simulink model "fw_att_control"  (R2024b)
settings: Solver=FixedStepAuto  StartTime=0.0  StopTime=10.0  FixedStep=0.005  RelTol=1e-3
undefined symbols (not defined in the file): DiscIntNeverNeededParam, FW_ACRO_X_MAX, FW_ACRO_Y_MAX, FW_ACRO_Z_MAX, FW_AIRSPD_MAX, FW_AIRSPD_STALL, FW_AIRSPD_TRIM, FW_ARSP_MODE, FW_ARSP_SCALE_EN, FW_BAT_SCALE_EN, FW_DTRIM_P_VMAX, FW_DTRIM_P_VMIN, FW_DTRIM_R_VMAX, FW_DTRIM_R_VMIN, FW_DTRIM_Y_VMAX, FW_DTRIM_Y_VMIN, FW_FLAPERON_SCL, FW_FLAPS_LND_SCL, FW_FLAPS_SCL, FW_FLAPS_TO_SCL, FW_MAN_P_MAX, FW_MAN_P_SC, FW_MAN_R_MAX, FW_MAN_R_SC, FW_MAN_Y_SC, FW_P_RMAX_NEG, FW_P_RMAX_POS, FW_P_TC, FW_PR_FF, FW_PR_IMAX, FW_PR_P, FW_PSP_OFF, FW_R_RMAX, FW_R_TC, FW_RLL_TO_YAW_FF, FW_RR_FF, FW_RR_IMAX, FW_RR_P, FW_W_RMAX, FW_WR_FF, FW_WR_IMAX, FW_WR_P, FW_Y_RMAX, FW_YR_FF, FW_YR_IMAX, FW_YR_P, TRIM_PITCH, TRIM_ROLL, TRIM_YAW
libraries: aerolibconvert2 x5, sharedtransform x2
settings Model: DataDictionary=nextpilot_datadict.sldd  Creator=CETCA  LastModifiedBy=CETCA
settings OptimizationCC: DefaultUnderspecifiedDataType=single
settings DebuggingCC: ParamPrecisionLossAbsoluteDiffThreshold=eps

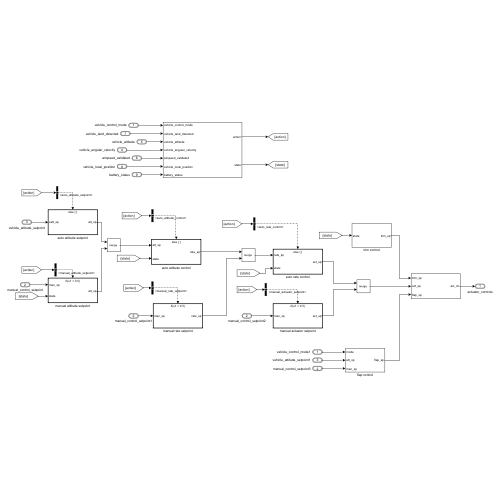
[thumbnail: Simulink's stored preview of the top-level diagram]
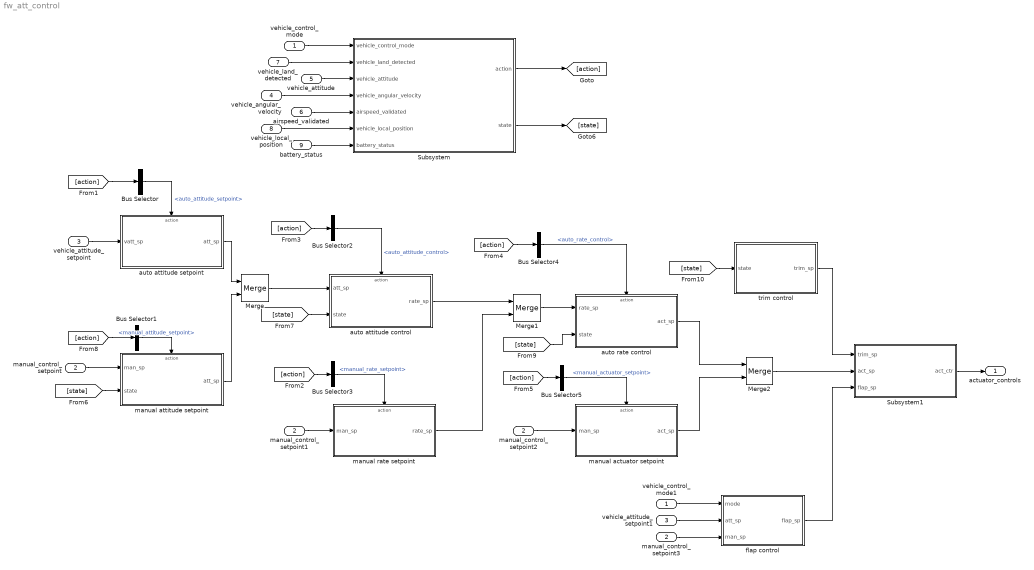
== system fw_att_control ==
  vehicle_control_mode : Inport  OutDataTypeStr=Bus: vehicle_control_mode_s
  manual_control_setpoint : Inport  Port=2  OutDataTypeStr=Bus: manual_control_setpoint_s
  vehicle_attitude_setpoint : Inport  Port=3  OutDataTypeStr=Bus:vehicle_attitude_setpoint_s
  vehicle_angular_velocity : Inport  Port=4  OutDataTypeStr=Bus: vehicle_angular_velocity_s
  vehicle_attitude : Inport  Port=5  OutDataTypeStr=Bus: vehicle_attitude_s
  airspeed_validated : Inport  Port=6  OutDataTypeStr=Bus: airspeed_validated_s
  vehicle_land_detected : Inport  Port=7  OutDataTypeStr=Bus: vehicle_land_detected_s
  vehicle_local_position : Inport  Port=8  OutDataTypeStr=Bus: vehicle_local_position_s
  battery_status : Inport  Port=9  OutDataTypeStr=Bus: battery_status_s
  Bus Selector : BusSelector  OutputSignals=auto_attitude_setpoint
  Bus Selector1 : BusSelector  OutputSignals=manual_attitude_setpoint
  Bus Selector2 : BusSelector  OutputSignals=auto_attitude_control
  Bus Selector3 : BusSelector  OutputSignals=manual_rate_setpoint
  Bus Selector4 : BusSelector  OutputSignals=auto_rate_control
  Bus Selector5 : BusSelector  OutputSignals=manual_actuator_setpoint
  Merge : Merge
  Merge1 : Merge
  Merge2 : Merge
  Subsystem : Subsystem
  Subsystem1 : Subsystem
  auto attitude control : Subsystem
  auto attitude setpoint : Subsystem
  auto rate control : Subsystem
  flap control : Subsystem
  manual actuator setpoint : Subsystem
  manual attitude setpoint : Subsystem
  manual rate setpoint : Subsystem
  manual_control_setpoint1 : InportShadow  Port=2  OutDataTypeStr=Bus: manual_control_setpoint_s
  manual_control_setpoint2 : InportShadow  Port=2  OutDataTypeStr=Bus: manual_control_setpoint_s
  manual_control_setpoint3 : InportShadow  Port=2  OutDataTypeStr=Bus: manual_control_setpoint_s
  trim control : Subsystem
  vehicle_attitude_setpoint1 : InportShadow  Port=3  OutDataTypeStr=Bus:vehicle_attitude_setpoint_s
  vehicle_control_mode1 : InportShadow  OutDataTypeStr=Bus: vehicle_control_mode_s
  actuator_controls : Outport  OutDataTypeStr=Bus: actuator_controls_s
  wires:
  manual_control_setpoint/1 -> manual attitude setpoint/1(man_sp)
  vehicle_attitude_setpoint/1 -> auto attitude setpoint/1(vatt_sp)
  Merge/1 -> auto attitude control/1(att_sp)
  auto attitude control/1(rate_sp) -> Merge1/1
  manual rate setpoint/1(rate_sp) -> Merge1/2
  Merge1/1 -> auto rate control/1(rate_sp)
  auto rate control/1(act_sp) -> Merge2/1
  manual actuator setpoint/1(act_sp) -> Merge2/2
  Bus Selector1/1 -> manual attitude setpoint/Action  "<manual_attitude_setpoint>"
  [action] -> Bus Selector/1
  Bus Selector3/1 -> manual rate setpoint/Action  "<manual_rate_setpoint>"
  Bus Selector2/1 -> auto attitude control/Action  "<auto_attitude_control>"
  Bus Selector5/1 -> manual actuator setpoint/Action  "<manual_actuator_setpoint>"
  Bus Selector4/1 -> auto rate control/Action  "<auto_rate_control>"
  vehicle_control_mode/1 -> Subsystem/1(vehicle_control_mode)
  manual_control_setpoint1/1 -> manual rate setpoint/1(man_sp)
  manual_control_setpoint2/1 -> manual actuator setpoint/1(man_sp)
  Subsystem/1(action) -> [action]
  vehicle_land_detected/1 -> Subsystem/2(vehicle_land_detected)
  airspeed_validated/1 -> Subsystem/5(airspeed_validated)
  vehicle_angular_velocity/1 -> Subsystem/4(vehicle_angular_velocity)
  vehicle_attitude/1 -> Subsystem/3(vehicle_attitude)
  Subsystem/2(state) -> [state]
  [state] -> manual attitude setpoint/2(state)
  vehicle_local_position/1 -> Subsystem/6(vehicle_local_position)
  [state] -> auto attitude control/2(state)
  manual attitude setpoint/1(att_sp) -> Merge/2
  auto attitude setpoint/1(att_sp) -> Merge/1
  Bus Selector/1 -> auto attitude setpoint/Action  "<auto_attitude_setpoint>"
  [action] -> Bus Selector1/1
  [action] -> Bus Selector2/1
  [action] -> Bus Selector3/1
  [action] -> Bus Selector4/1
  [action] -> Bus Selector5/1
  [state] -> auto rate control/2(state)
  battery_status/1 -> Subsystem/7(battery_status)
  Merge2/1 -> Subsystem1/2(act_sp)
  vehicle_attitude_setpoint1/1 -> flap control/2(att_sp)
  manual_control_setpoint3/1 -> flap control/3(man_sp)
  vehicle_control_mode1/1 -> flap control/1(mode)
  flap control/1(flap_sp) -> Subsystem1/3(flap_sp)
  Subsystem1/1(act_ctr) -> actuator_controls/1
  [state] -> trim control/1(state)
  trim control/1(trim_sp) -> Subsystem1/1(trim_sp)

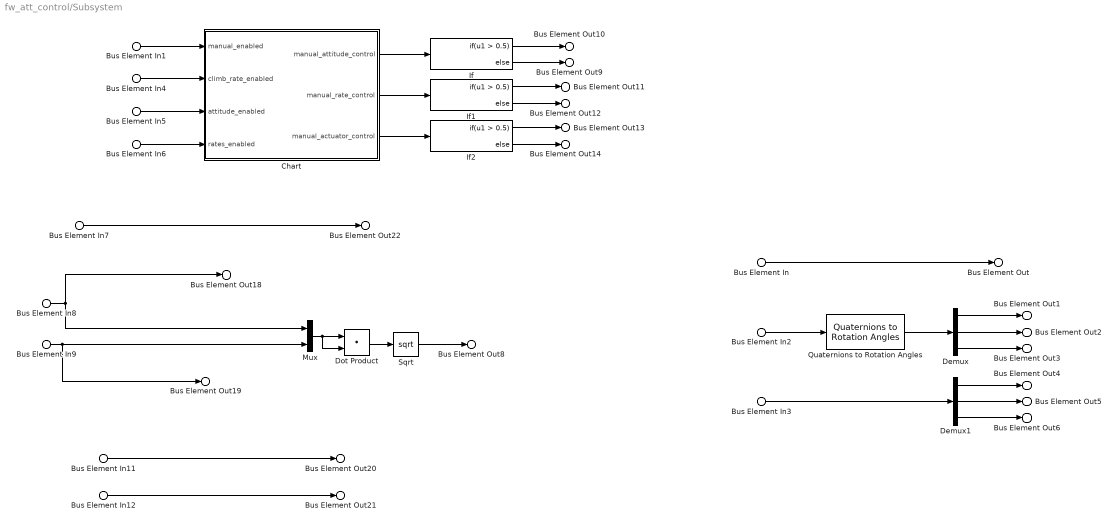
== system fw_att_control/Subsystem ==
  Bus Element In1 : Inport  PortName=vehicle_control_mode  Element=flag_control_manual_enabled
  Bus Element In4 : Inport  PortName=vehicle_control_mode  Element=flag_control_climb_rate_enabled
  Bus Element In5 : Inport  PortName=vehicle_control_mode  Element=flag_control_attitude_enabled
  Bus Element In6 : Inport  PortName=vehicle_control_mode  Element=flag_control_rates_enabled
  Bus Element In : Inport  Port=2  PortName=vehicle_land_detected  Element=landed
  Bus Element In2 : Inport  Port=3  PortName=vehicle_attitude  Element=q
  Bus Element In3 : Inport  Port=4  PortName=vehicle_angular_velocity  Element=xyz
  Bus Element In7 : Inport  Port=5  PortName=airspeed_validated  Element=calibrated_airspeed_m_s
  Bus Element In8 : Inport  Port=6  PortName=vehicle_local_position  Element=vx
  Bus Element In9 : Inport  Port=6  PortName=vehicle_local_position  Element=vy
  Bus Element In11 : Inport  Port=7  PortName=battery_status  Element=connected
  Bus Element In12 : Inport  Port=7  PortName=battery_status  Element=scale
  Chart : Stateflow chart  TreatAsAtomicUnit=on
  Demux : Demux  Outputs=3
  Demux1 : Demux  Outputs=3
  Dot Product : DotProduct  OutDataTypeStr=Inherit: Inherit via internal rule
  If : If  IfExpression=u1 > 0.5
  If1 : If  IfExpression=u1 > 0.5
  If2 : If  IfExpression=u1 > 0.5
  Mux : Mux  Inputs=2
  Quaternions to Rotation Angles : sharedtransform/Quaternions to Rotation Angles  rotationOrder=ZYX  aMode=aMode
  Sqrt : Sqrt
  Bus Element Out10 : Outport  PortName=action  Element=manual_attitude_setpoint
  Bus Element Out9 : Outport  PortName=action  Element=auto_attitude_setpoint
  Bus Element Out11 : Outport  PortName=action  Element=manual_rate_setpoint
  Bus Element Out12 : Outport  PortName=action  Element=auto_attitude_control
  Bus Element Out13 : Outport  PortName=action  Element=manual_actuator_setpoint
  Bus Element Out14 : Outport  PortName=action  Element=auto_rate_control
  Bus Element Out : Outport  Port=2  PortName=state  Element=landed
  Bus Element Out1 : Outport  Port=2  PortName=state  Element=yaw
  Bus Element Out2 : Outport  Port=2  PortName=state  Element=pitch
  Bus Element Out3 : Outport  Port=2  PortName=state  Element=roll
  Bus Element Out4 : Outport  Port=2  PortName=state  Element=roll_speed
  Bus Element Out5 : Outport  Port=2  PortName=state  Element=pitch_speed
  Bus Element Out6 : Outport  Port=2  PortName=state  Element=yaw_speed
  Bus Element Out8 : Outport  Port=2  PortName=state  Element=groud_speed
  Bus Element Out18 : Outport  Port=2  PortName=state  Element=north_speed
  Bus Element Out19 : Outport  Port=2  PortName=state  Element=east_speed
  Bus Element Out20 : Outport  Port=2  PortName=state  Element=battery.connected
  Bus Element Out21 : Outport  Port=2  PortName=state  Element=battery.scale
  Bus Element Out22 : Outport  Port=2  PortName=state  Element=calibrated_airspeed
  wires:
  Chart/1(manual_attitude_control) -> If/1
  If/1 -> Bus Element Out10/1
  Bus Element In1/1 -> Chart/1(manual_enabled)
  If2/2 -> Bus Element Out14/1
  Chart/3(manual_actuator_control) -> If2/1
  If/2 -> Bus Element Out9/1
  If1/1 -> Bus Element Out11/1
  Chart/2(manual_rate_control) -> If1/1
  If1/2 -> Bus Element Out12/1
  Bus Element In4/1 -> Chart/2(climb_rate_enabled)
  If2/1 -> Bus Element Out13/1
  Bus Element In5/1 -> Chart/3(attitude_enabled)
  Bus Element In6/1 -> Chart/4(rates_enabled)
  Demux/1 -> Bus Element Out1/1
  Demux1/1 -> Bus Element Out4/1
  Bus Element In3/1 -> Demux1/1
  Bus Element In/1 -> Bus Element Out/1
  Quaternions to Rotation Angles/1 -> Demux/1
  Demux/2 -> Bus Element Out2/1
  Demux/3 -> Bus Element Out3/1
  Demux1/2 -> Bus Element Out5/1
  Demux1/3 -> Bus Element Out6/1
  Bus Element In2/1 -> Quaternions to Rotation Angles/1
  Bus Element In7/1 -> Bus Element Out22/1
  Bus Element In8/1 -> Mux/1, Bus Element Out18/1
  Bus Element In9/1 -> Mux/2, Bus Element Out19/1
  Bus Element In11/1 -> Bus Element Out20/1
  Bus Element In12/1 -> Bus Element Out21/1
  Sqrt/1 -> Bus Element Out8/1
  Mux/1 -> Dot Product/2, Dot Product/1
  Dot Product/1 -> Sqrt/1

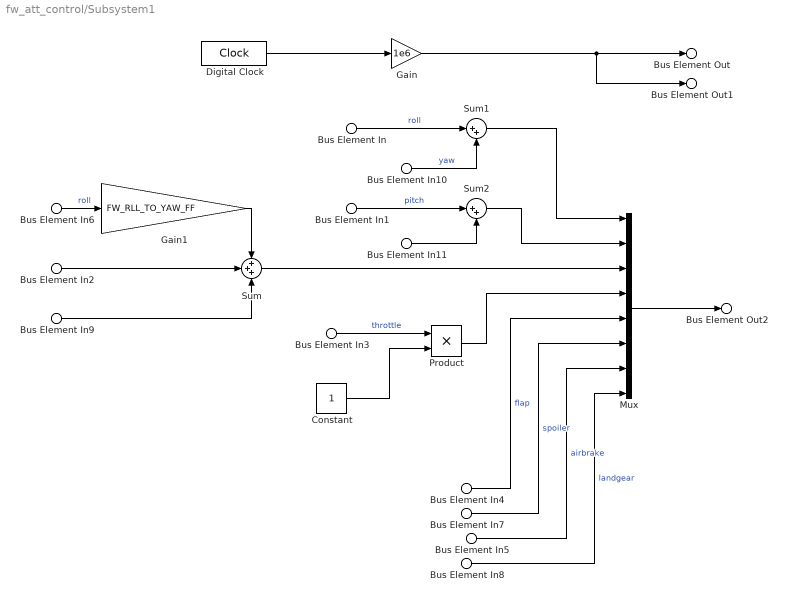
== system fw_att_control/Subsystem1 ==
  Bus Element In9 : Inport  PortName=trim_sp  Element=yaw
  Bus Element In10 : Inport  PortName=trim_sp  Element=roll
  Bus Element In11 : Inport  PortName=trim_sp  Element=pitch
  Bus Element In : Inport  Port=2  PortName=act_sp  Element=roll
  Bus Element In6 : Inport  Port=2  PortName=act_sp  Element=roll
  Bus Element In1 : Inport  Port=2  PortName=act_sp  Element=pitch
  Bus Element In2 : Inport  Port=2  PortName=act_sp  Element=yaw
  Bus Element In3 : Inport  Port=2  PortName=act_sp  Element=throttle
  Bus Element In4 : Inport  Port=3  PortName=flap_sp  Element=flap
  Bus Element In5 : Inport  Port=3  PortName=flap_sp  Element=flaperon
  Bus Element In7 : Inport  Port=3  PortName=flap_sp  Element=aux1
  Bus Element In8 : Inport  Port=3  PortName=flap_sp  Element=aux3
  Constant : Constant  OutDataTypeStr=single
  Digital Clock : DigitalClock  SampleTime=-1
  Gain : Gain  Gain=1e6  OutDataTypeStr=uint64
  Gain1 : Gain  Gain=FW_RLL_TO_YAW_FF  OutDataTypeStr=uint64
  Mux : Mux  Inputs=8
  Product : Product
  Sum : Sum  Inputs=3
  Sum1 : Sum  Inputs=|++
  Sum2 : Sum  Inputs=|++
  Bus Element Out : Outport  PortName=act_ctr  Element=timestamp
  Bus Element Out1 : Outport  PortName=act_ctr  Element=timestamp_sample
  Bus Element Out2 : Outport  PortName=act_ctr  Element=control
  wires:
  Bus Element In/1 -> Sum1/1  "roll"
  Bus Element In1/1 -> Sum2/1  "pitch"
  Bus Element In3/1 -> Product/1  "throttle"
  Digital Clock/1 -> Gain/1
  Gain/1 -> Bus Element Out1/1, Bus Element Out/1
  Mux/1 -> Bus Element Out2/1
  Bus Element In4/1 -> Mux/5  "flap"
  Bus Element In5/1 -> Mux/7  "airbrake"
  Bus Element In8/1 -> Mux/8  "landgear"
  Bus Element In7/1 -> Mux/6  "spoiler"
  Bus Element In6/1 -> Gain1/1  "roll"
  Sum/1 -> Mux/3
  Bus Element In2/1 -> Sum/2
  Gain1/1 -> Sum/1
  Bus Element In9/1 -> Sum/3
  Bus Element In10/1 -> Sum1/2  "yaw"
  Sum1/1 -> Mux/1
  Sum2/1 -> Mux/2
  Bus Element In11/1 -> Sum2/2
  Product/1 -> Mux/4
  Constant/1 -> Product/2

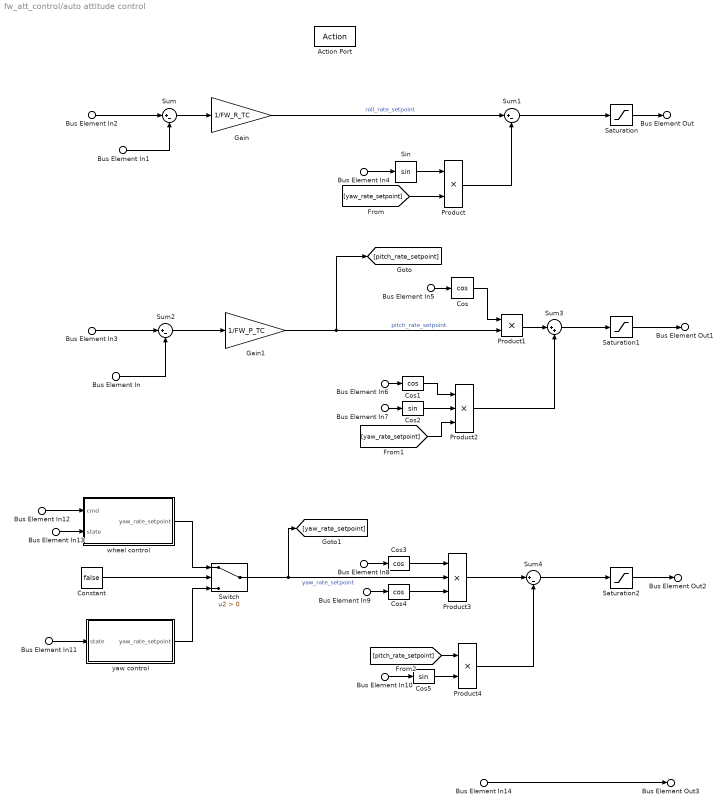
== system fw_att_control/auto attitude control ==
  Bus Element In12 : Inport  PortName=att_sp
  Bus Element In2 : Inport  PortName=att_sp  Element=roll_body
  Bus Element In3 : Inport  PortName=att_sp  Element=pitch_body
  Bus Element In14 : Inport  PortName=att_sp  Element=thrust_body
  Bus Element In11 : Inport  Port=2  PortName=state
  Bus Element In13 : Inport  Port=2  PortName=state
  Bus Element In{,4,6,9} (4 alike) : Inport  Port=2  PortName=state  Element=pitch
  Bus Element In{1,5,7..8,10} (5 alike) : Inport  Port=2  PortName=state  Element=roll
  Action Port : ActionPort  ActionPortLabel=else
  Constant : Constant  Value=false
  Cos{,1,3..4} (4 alike) : Trigonometry  Operator=cos
  Cos2 : Trigonometry
  Cos5 : Trigonometry
  Gain : Gain  Gain=1/FW_R_TC
  Gain1 : Gain  Gain=1/FW_P_TC
  Product : Product
  Product1 : Product
  Product2 : Product  Inputs=3
  Product3 : Product  Inputs=3
  Product4 : Product
  Saturation : Saturate  UpperLimit=FW_R_RMAX  LowerLimit=-FW_R_RMAX
  Saturation1 : Saturate  UpperLimit=FW_P_RMAX_POS  LowerLimit=-FW_P_RMAX_NEG
  Saturation2 : Saturate  UpperLimit=FW_Y_RMAX  LowerLimit=-FW_Y_RMAX
  Sin : Trigonometry
  Sum{,1..2,4} (4 alike) : Sum  Inputs=|+-
  Sum3 : Sum  Inputs=|++
  Switch : Switch  Criteria=u2 > Threshold  SaturateOnIntegerOverflow=off  InputSameDT=off
  wheel control : Subsystem
  yaw control : Subsystem
  Bus Element Out : Outport  PortName=rate_sp  Element=roll
  Bus Element Out1 : Outport  PortName=rate_sp  Element=pitch
  Bus Element Out2 : Outport  PortName=rate_sp  Element=yaw
  Bus Element Out3 : Outport  PortName=rate_sp  Element=thrust_body
  wires:
  Switch/1 -> [yaw_rate_setpoint], Product3/2  "yaw_rate_setpoint"
  Bus Element In11/1 -> yaw control/1(state)
  Bus Element In12/1 -> wheel control/1(cmd)
  Cos3/1 -> Product3/1
  Sin/1 -> Product/1
  wheel control/1(yaw_rate_setpoint) -> Switch/1
  Sum1/1 -> Saturation/1
  Cos4/1 -> Product3/3
  Gain1/1 -> [pitch_rate_setpoint], Product1/2  "pitch_rate_setpoint"
  Bus Element In8/1 -> Cos3/1
  Cos2/1 -> Product2/2
  Product4/1 -> Sum4/2
  Cos5/1 -> Product4/2
  [pitch_rate_setpoint] -> Product4/1
  Product3/1 -> Sum4/1
  Product/1 -> Sum1/2
  Cos/1 -> Product1/1
  Bus Element In10/1 -> Cos5/1
  Sum4/1 -> Saturation2/1
  Saturation/1 -> Bus Element Out/1
  Sum2/1 -> Gain1/1
  [yaw_rate_setpoint] -> Product/2
  Saturation2/1 -> Bus Element Out2/1
  Bus Element In/1 -> Sum2/2
  Bus Element In7/1 -> Cos2/1
  Gain/1 -> Sum1/1  "roll_rate_setpoint"
  Bus Element In1/1 -> Sum/2
  Bus Element In5/1 -> Cos/1
  Sum3/1 -> Saturation1/1
  Sum/1 -> Gain/1
  Bus Element In6/1 -> Cos1/1
  Bus Element In4/1 -> Sin/1
  Product2/1 -> Sum3/2
  Constant/1 -> Switch/2
  [yaw_rate_setpoint] -> Product2/3
  Bus Element In2/1 -> Sum/1
  Bus Element In9/1 -> Cos4/1
  Product1/1 -> Sum3/1
  Cos1/1 -> Product2/1
  Bus Element In13/1 -> wheel control/2(state)
  Bus Element In3/1 -> Sum2/1
  Saturation1/1 -> Bus Element Out1/1
  yaw control/1(yaw_rate_setpoint) -> Switch/3
  Bus Element In14/1 -> Bus Element Out3/1

== system fw_att_control/auto attitude setpoint ==
  vatt_sp : Inport
  Action Port : ActionPort  ActionPortLabel=else
  To Virtual Bus : SignalConversion  Commented=through  ConversionOutput=Virtual bus  OverrideOpt=off
  att_sp : Outport
  wires:
  To Virtual Bus/1 -> att_sp/1
  vatt_sp/1 -> To Virtual Bus/1

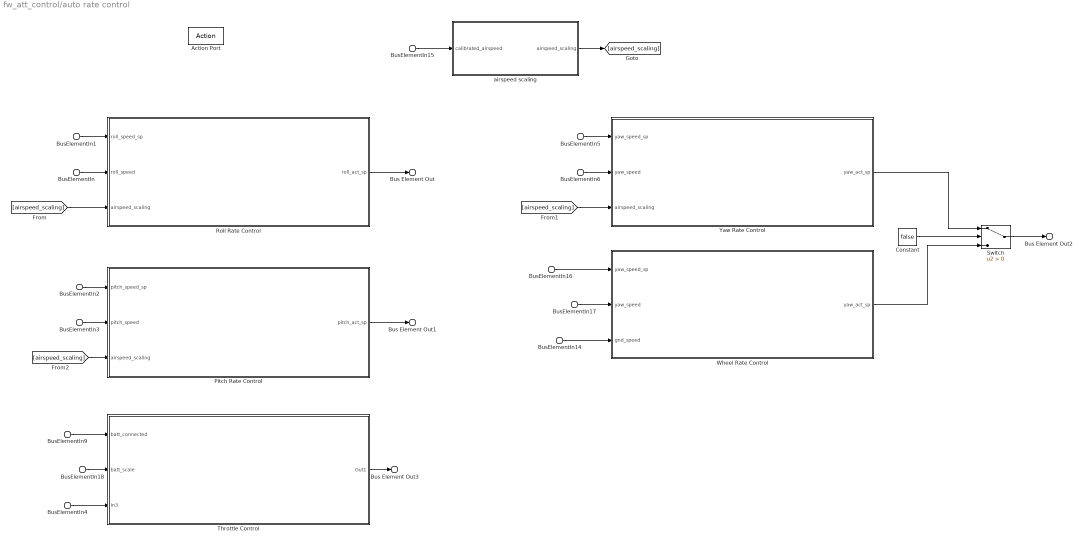
== system fw_att_control/auto rate control ==
  BusElementIn1 : Inport  PortName=rate_sp  Element=roll
  BusElementIn2 : Inport  PortName=rate_sp  Element=pitch
  BusElementIn4 : Inport  PortName=rate_sp  Element=thrust_body
  BusElementIn5 : Inport  PortName=rate_sp  Element=yaw
  BusElementIn16 : Inport  PortName=rate_sp  Element=yaw
  BusElementIn : Inport  Port=2  PortName=state  Element=roll_speed
  BusElementIn3 : Inport  Port=2  PortName=state  Element=pitch_speed
  BusElementIn6 : Inport  Port=2  PortName=state  Element=yaw_speed
  BusElementIn17 : Inport  Port=2  PortName=state  Element=yaw_speed
  BusElementIn14 : Inport  Port=2  PortName=state  Element=groud_speed
  BusElementIn15 : Inport  Port=2  PortName=state  Element=calibrated_airspeed
  BusElementIn9 : Inport  Port=2  PortName=state  Element=battery.connected
  BusElementIn18 : Inport  Port=2  PortName=state  Element=battery.scale
  Action Port : ActionPort  ActionPortLabel=else
  Constant : Constant  Value=false
  Pitch Rate Control : Subsystem
  Roll Rate Control : Subsystem
  Switch : Switch  Criteria=u2 > Threshold  SaturateOnIntegerOverflow=off  InputSameDT=off
  Throttle Control : Subsystem
  Wheel Rate Control : Subsystem
  Yaw Rate Control : Subsystem
  airspeed scaling : Subsystem
  Bus Element Out : Outport  PortName=act_sp  Element=roll
  Bus Element Out1 : Outport  PortName=act_sp  Element=pitch
  Bus Element Out2 : Outport  PortName=act_sp  Element=yaw
  Bus Element Out3 : Outport  PortName=act_sp  Element=throttle
  wires:
  BusElementIn1/1 -> Roll Rate Control/1(roll_speed_sp)
  BusElementIn/1 -> Roll Rate Control/2(roll_speed)
  Roll Rate Control/1(roll_act_sp) -> Bus Element Out/1
  BusElementIn2/1 -> Pitch Rate Control/1(pitch_speed_sp)
  BusElementIn3/1 -> Pitch Rate Control/2(pitch_speed)
  Pitch Rate Control/1(pitch_act_sp) -> Bus Element Out1/1
  Yaw Rate Control/1(yaw_act_sp) -> Switch/1
  BusElementIn5/1 -> Yaw Rate Control/1(yaw_speed_sp)
  BusElementIn6/1 -> Yaw Rate Control/2(yaw_speed)
  [airspeed_scaling] -> Pitch Rate Control/3(airspeed_scaling)
  BusElementIn14/1 -> Wheel Rate Control/3(gnd_speed)
  BusElementIn15/1 -> airspeed scaling/1(calibrated_airspeed)
  BusElementIn16/1 -> Wheel Rate Control/1(yaw_speed_sp)
  BusElementIn17/1 -> Wheel Rate Control/2(yaw_speed)
  BusElementIn9/1 -> Throttle Control/1(batt_connected)
  BusElementIn18/1 -> Throttle Control/2(batt_scale)
  BusElementIn4/1 -> Throttle Control/3(In3)
  Throttle Control/1(Out1) -> Bus Element Out3/1
  airspeed scaling/1(airspeed_scaling) -> [airspeed_scaling]
  [airspeed_scaling] -> Roll Rate Control/3(airspeed_scaling)
  [airspeed_scaling] -> Yaw Rate Control/3(airspeed_scaling)
  Wheel Rate Control/1(yaw_act_sp) -> Switch/3
  Switch/1 -> Bus Element Out2/1
  Constant/1 -> Switch/2

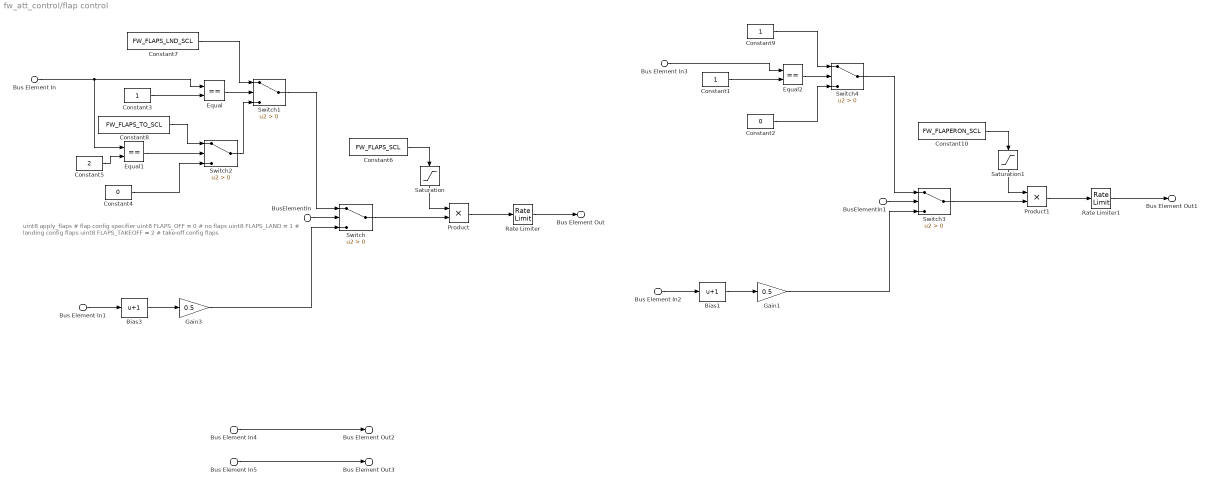
== system fw_att_control/flap control ==
  note: uint8 apply_flaps       	# flap config specifier
      | uint8 FLAPS_OFF = 0     	# no flaps
      | uint8 FLAPS_LAND = 1    	# landing config flaps
      | uint8 FLAPS_TAKEOFF = 2 	# take-off config flaps
  BusElementIn : Inport  PortName=mode  Element=flag_control_auto_enabled
  BusElementIn1 : Inport  PortName=mode  Element=flag_control_auto_enabled
  Bus Element In : Inport  Port=2  PortName=att_sp  Element=apply_flaps
  Bus Element In3 : Inport  Port=2  PortName=att_sp  Element=apply_flaps
  Bus Element In1 : Inport  Port=3  PortName=man_sp  Element=flaps
  Bus Element In2 : Inport  Port=3  PortName=man_sp  Element=aux2
  Bus Element In4 : Inport  Port=3  PortName=man_sp  Element=aux1
  Bus Element In5 : Inport  Port=3  PortName=man_sp  Element=aux3
  Bias1 : Bias  Bias=1  SaturateOnIntegerOverflow=off
  Bias3 : Bias  Bias=1  SaturateOnIntegerOverflow=off
  Constant1 : Constant  OutDataTypeStr=single
  Constant10 : Constant  Value=FW_FLAPERON_SCL
  Constant2 : Constant  Value=0  OutDataTypeStr=single
  Constant3 : Constant  OutDataTypeStr=single
  Constant4 : Constant  Value=0  OutDataTypeStr=single
  Constant5 : Constant  Value=2  OutDataTypeStr=single
  Constant6 : Constant  Value=FW_FLAPS_SCL
  Constant7 : Constant  Value=FW_FLAPS_LND_SCL
  Constant8 : Constant  Value=FW_FLAPS_TO_SCL
  Constant9 : Constant  OutDataTypeStr=single
  Equal : RelationalOperator  Operator===  OutDataTypeStr=boolean  RndMeth=Simplest  InputSameDT=off
  Equal1 : RelationalOperator  Operator===  OutDataTypeStr=boolean  RndMeth=Simplest  InputSameDT=off
  Equal2 : RelationalOperator  Operator===  OutDataTypeStr=boolean  RndMeth=Simplest  InputSameDT=off
  Gain1 : Gain  Gain=0.5
  Gain3 : Gain  Gain=0.5
  Product : Product
  Product1 : Product
  Rate Limiter : RateLimiter  SampleTimeMode=inherited
  Rate Limiter1 : RateLimiter  SampleTimeMode=inherited
  Saturation : Saturate  UpperLimit=1  LowerLimit=0
  Saturation1 : Saturate  UpperLimit=1  LowerLimit=0
  Switch{,1..4} (5 alike) : Switch  Criteria=u2 > Threshold  SaturateOnIntegerOverflow=off  InputSameDT=off
  Bus Element Out : Outport  PortName=flap_sp  Element=flap
  Bus Element Out1 : Outport  PortName=flap_sp  Element=flaperon
  Bus Element Out2 : Outport  PortName=flap_sp  Element=aux1
  Bus Element Out3 : Outport  PortName=flap_sp  Element=aux3
  wires:
  Equal/1 -> Switch1/2
  Gain3/1 -> Switch/3
  Switch1/1 -> Switch/1
  Saturation/1 -> Product/1
  Constant8/1 -> Switch2/1
  Constant3/1 -> Equal/2
  Bias3/1 -> Gain3/1
  Switch/1 -> Product/2
  Bus Element In/1 -> Equal1/1, Equal/1
  Constant6/1 -> Saturation/1
  Equal1/1 -> Switch2/2
  BusElementIn/1 -> Switch/2
  Switch2/1 -> Switch1/3
  Constant7/1 -> Switch1/1
  Constant4/1 -> Switch2/3
  Constant5/1 -> Equal1/2
  Bus Element In1/1 -> Bias3/1
  Product/1 -> Rate Limiter/1
  Rate Limiter/1 -> Bus Element Out/1
  BusElementIn1/1 -> Switch3/2
  Bus Element In3/1 -> Equal2/1
  Constant2/1 -> Switch4/3
  Saturation1/1 -> Product1/1
  Gain1/1 -> Switch3/3
  Equal2/1 -> Switch4/2
  Constant10/1 -> Saturation1/1
  Constant9/1 -> Switch4/1
  Switch3/1 -> Product1/2
  Rate Limiter1/1 -> Bus Element Out1/1
  Constant1/1 -> Equal2/2
  Bias1/1 -> Gain1/1
  Bus Element In2/1 -> Bias1/1
  Switch4/1 -> Switch3/1
  Product1/1 -> Rate Limiter1/1
  Bus Element In4/1 -> Bus Element Out2/1
  Bus Element In5/1 -> Bus Element Out3/1

== system fw_att_control/manual actuator setpoint ==
  Bus Element In : Inport  PortName=man_sp  Element=y
  Bus Element In1 : Inport  PortName=man_sp  Element=x
  Bus Element In2 : Inport  PortName=man_sp  Element=r
  Bus Element In4 : Inport  PortName=man_sp  Element=z
  Action Port : ActionPort  ActionPortLabel=if(u1 > 0.5)
  Bias : Bias  Bias=TRIM_ROLL  SaturateOnIntegerOverflow=off
  Bias1 : Bias  Bias=TRIM_PITCH  SaturateOnIntegerOverflow=off
  Bias2 : Bias  Bias=TRIM_YAW  SaturateOnIntegerOverflow=off
  Gain : Gain  Gain=FW_MAN_R_SC
  Gain1 : Gain  Gain=-FW_MAN_P_SC
  Gain2 : Gain  Gain=FW_MAN_Y_SC
  Saturation1 : Saturate  UpperLimit=1  LowerLimit=0
  Bus Element Out3 : Outport  PortName=act_sp  Element=roll
  Bus Element Out1 : Outport  PortName=act_sp  Element=pitch
  Bus Element Out2 : Outport  PortName=act_sp  Element=yaw
  Bus Element Out4 : Outport  PortName=act_sp  Element=throttle
  wires:
  Bus Element In2/1 -> Gain2/1
  Bus Element In/1 -> Gain/1
  Bus Element In1/1 -> Gain1/1
  Gain/1 -> Bias/1
  Gain1/1 -> Bias1/1
  Gain2/1 -> Bias2/1
  Bus Element In4/1 -> Saturation1/1
  Bias2/1 -> Bus Element Out2/1
  Bias1/1 -> Bus Element Out1/1
  Bias/1 -> Bus Element Out3/1
  Saturation1/1 -> Bus Element Out4/1

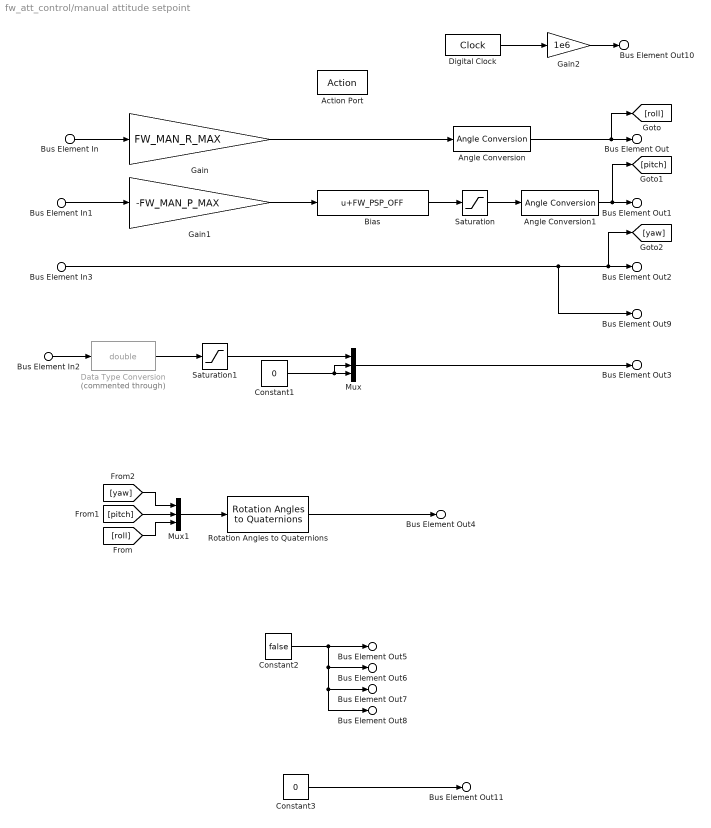
== system fw_att_control/manual attitude setpoint ==
  Bus Element In : Inport  PortName=man_sp  Element=y
  Bus Element In1 : Inport  PortName=man_sp  Element=x
  Bus Element In2 : Inport  PortName=man_sp  Element=z
  Bus Element In3 : Inport  Port=2  PortName=state  Element=yaw
  Action Port : ActionPort  ActionPortLabel=if(u1 > 0.5)
  Angle Conversion : aerolibconvert2/Angle Conversion  IU=deg  OU=rad
  Angle Conversion1 : aerolibconvert2/Angle Conversion  IU=deg  OU=rad
  Bias : Bias  Bias=FW_PSP_OFF  SaturateOnIntegerOverflow=off
  Constant1 : Constant  Value=0  OutDataTypeStr=single
  Constant2 : Constant  Value=false
  Constant3 : Constant  Value=0  OutDataTypeStr=uint8
  Data Type Conversion : DataTypeConversion  Commented=through  OutDataTypeStr=double  SaturateOnIntegerOverflow=off  RndMeth=Floor
  Digital Clock : DigitalClock  SampleTime=-1
  Gain : Gain  Gain=FW_MAN_R_MAX
  Gain1 : Gain  Gain=-FW_MAN_P_MAX
  Gain2 : Gain  Gain=1e6  ParamDataTypeStr=uint64  OutDataTypeStr=uint64
  Mux : Mux  Inputs=3
  Mux1 : Mux  Inputs=3
  Rotation Angles to Quaternions : sharedtransform/Rotation Angles to Quaternions  rotationOrder=ZYX  aMode=aMode
  Saturation : Saturate  UpperLimit=FW_MAN_P_MAX  LowerLimit=-FW_MAN_P_MAX
  Saturation1 : Saturate  UpperLimit=1  LowerLimit=0
  Bus Element Out10 : Outport  PortName=att_sp  Element=timestamp
  Bus Element Out : Outport  PortName=att_sp  Element=roll_body
  Bus Element Out1 : Outport  PortName=att_sp  Element=pitch_body
  Bus Element Out2 : Outport  PortName=att_sp  Element=yaw_body
  Bus Element Out9 : Outport  PortName=att_sp  Element=yaw_sp_move_rate
  Bus Element Out4 : Outport  PortName=att_sp  Element=q_d
  Bus Element Out3 : Outport  PortName=att_sp  Element=thrust_body
  Bus Element Out5 : Outport  PortName=att_sp  Element=roll_reset_integral
  Bus Element Out6 : Outport  PortName=att_sp  Element=pitch_reset_integral
  Bus Element Out7 : Outport  PortName=att_sp  Element=yaw_reset_integral
  Bus Element Out8 : Outport  PortName=att_sp  Element=fw_control_yaw
  Bus Element Out11 : Outport  PortName=att_sp  Element=apply_flaps
  wires:
  Bus Element In/1 -> Gain/1
  Gain/1 -> Angle Conversion/1
  Bus Element In1/1 -> Gain1/1
  Gain1/1 -> Bias/1
  Bias/1 -> Saturation/1
  Saturation/1 -> Angle Conversion1/1
  Bus Element In3/1 -> Bus Element Out9/1, [yaw], Bus Element Out2/1
  Mux/1 -> Bus Element Out3/1
  Constant1/1 -> Mux/2, Mux/3
  Bus Element In2/1 -> Data Type Conversion/1
  Saturation1/1 -> Mux/1
  Angle Conversion/1 -> [roll], Bus Element Out/1
  Angle Conversion1/1 -> [pitch], Bus Element Out1/1
  [pitch] -> Mux1/2
  [yaw] -> Mux1/1
  [roll] -> Mux1/3
  Mux1/1 -> Rotation Angles to Quaternions/1
  Rotation Angles to Quaternions/1 -> Bus Element Out4/1
  Constant2/1 -> Bus Element Out8/1, Bus Element Out7/1, Bus Element Out6/1, Bus Element Out5/1
  Data Type Conversion/1 -> Saturation1/1
  Digital Clock/1 -> Gain2/1
  Gain2/1 -> Bus Element Out10/1
  Constant3/1 -> Bus Element Out11/1

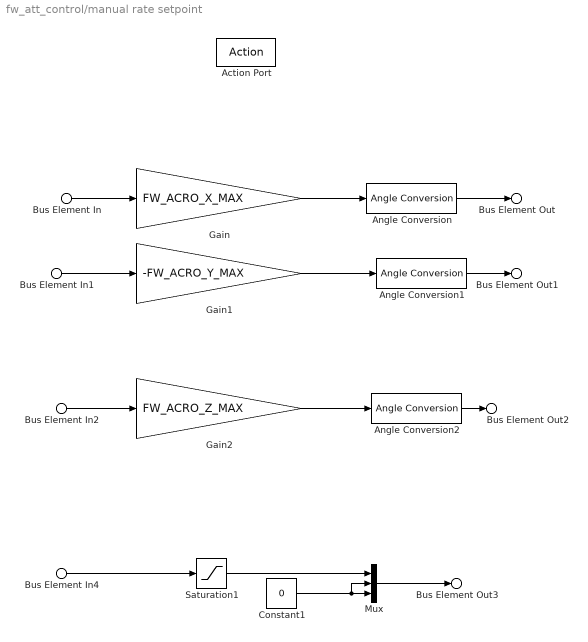
== system fw_att_control/manual rate setpoint ==
  Bus Element In : Inport  PortName=man_sp  Element=y
  Bus Element In1 : Inport  PortName=man_sp  Element=x
  Bus Element In2 : Inport  PortName=man_sp  Element=r
  Bus Element In4 : Inport  PortName=man_sp  Element=z
  Action Port : ActionPort  ActionPortLabel=if(u1 > 0.5)
  Angle Conversion : aerolibconvert2/Angle Conversion  IU=deg  OU=rad
  Angle Conversion1 : aerolibconvert2/Angle Conversion  IU=deg  OU=rad
  Angle Conversion2 : aerolibconvert2/Angle Conversion  IU=deg  OU=rad
  Constant1 : Constant  Value=0  OutDataTypeStr=single
  Gain : Gain  Gain=FW_ACRO_X_MAX
  Gain1 : Gain  Gain=-FW_ACRO_Y_MAX
  Gain2 : Gain  Gain=FW_ACRO_Z_MAX
  Mux : Mux  Inputs=3
  Saturation1 : Saturate  UpperLimit=1  LowerLimit=0
  Bus Element Out : Outport  PortName=rate_sp  Element=roll
  Bus Element Out1 : Outport  PortName=rate_sp  Element=pitch
  Bus Element Out2 : Outport  PortName=rate_sp  Element=yaw
  Bus Element Out3 : Outport  PortName=rate_sp  Element=thrust_body
  wires:
  Bus Element In2/1 -> Gain2/1
  Bus Element In/1 -> Gain/1
  Bus Element In1/1 -> Gain1/1
  Gain/1 -> Angle Conversion/1
  Gain1/1 -> Angle Conversion1/1
  Gain2/1 -> Angle Conversion2/1
  Bus Element In4/1 -> Saturation1/1
  Mux/1 -> Bus Element Out3/1
  Constant1/1 -> Mux/2, Mux/3
  Saturation1/1 -> Mux/1
  Angle Conversion/1 -> Bus Element Out/1
  Angle Conversion1/1 -> Bus Element Out1/1
  Angle Conversion2/1 -> Bus Element Out2/1

== system fw_att_control/trim control ==
  Bus Element In : Inport  PortName=state  Element=calibrated_airspeed
  Bus Element In1 : Inport  PortName=state  Element=calibrated_airspeed
  Bus Element In2 : Inport  PortName=state  Element=calibrated_airspeed
  1-D Lookup Table : Lookup_n-D  NumberOfTableDimensions=1  BreakpointsForDimension1=[FW_AIRSPD_STALL, FW_AIRSPD_TRIM, FW_AIRSPD_MAX]  IndexSearchMethod=Linear search  BeginIndexSearchUsingPreviousIndexResult=on  Table=[FW_DTRIM_Y_VMIN, 0, FW_DTRIM_Y_VMAX]  ExtrapMethod=Clip  InternalRulePriority=Speed  RndMeth=Simplest
  1-D Lookup Table1 : Lookup_n-D  NumberOfTableDimensions=1  BreakpointsForDimension1=[FW_AIRSPD_STALL, FW_AIRSPD_TRIM, FW_AIRSPD_MAX]  IndexSearchMethod=Linear search  BeginIndexSearchUsingPreviousIndexResult=on  Table=[FW_DTRIM_R_VMIN, 0, FW_DTRIM_R_VMAX]  ExtrapMethod=Clip  InternalRulePriority=Speed  RndMeth=Simplest
  1-D Lookup Table2 : Lookup_n-D  NumberOfTableDimensions=1  BreakpointsForDimension1=[FW_AIRSPD_STALL, FW_AIRSPD_TRIM, FW_AIRSPD_MAX]  IndexSearchMethod=Linear search  BeginIndexSearchUsingPreviousIndexResult=on  Table=[FW_DTRIM_P_VMIN, 0, FW_DTRIM_P_VMAX]  ExtrapMethod=Clip  InternalRulePriority=Speed  RndMeth=Simplest
  Constant1 : Constant  Value=TRIM_ROLL
  Constant2 : Constant  Value=TRIM_PITCH
  Constant5 : Constant  Value=TRIM_YAW
  Sum1 : Sum  Inputs=|++
  Sum2 : Sum  Inputs=|++
  Sum3 : Sum  Inputs=|++
  Bus Element Out : Outport  PortName=trim_sp  Element=yaw
  Bus Element Out1 : Outport  PortName=trim_sp  Element=roll
  Bus Element Out2 : Outport  PortName=trim_sp  Element=pitch
  wires:
  Constant5/1 -> Sum1/1
  Sum1/1 -> Bus Element Out/1
  1-D Lookup Table/1 -> Sum1/2
  Bus Element In/1 -> 1-D Lookup Table/1
  Constant1/1 -> Sum2/1
  1-D Lookup Table1/1 -> Sum2/2
  Bus Element In1/1 -> 1-D Lookup Table1/1
  Sum2/1 -> Bus Element Out1/1
  Constant2/1 -> Sum3/1
  1-D Lookup Table2/1 -> Sum3/2
  Sum3/1 -> Bus Element Out2/1
  Bus Element In2/1 -> 1-D Lookup Table2/1

== system fw_att_control/auto attitude control/wheel control ==
  Bus Element In : Inport  PortName=cmd  Element=yaw_body
  Bus Element In1 : Inport  Port=2  PortName=state  Element=yaw
  Constant : Constant  Value=single(2*pi)  OutDataTypeStr=single
  Gain : Gain  Gain=1/0.1
  Mod : Math  Operator=mod
  Saturation : Saturate  UpperLimit=FW_W_RMAX  LowerLimit=-FW_W_RMAX
  Sum : Sum  Inputs=|+-
  Sum1 : Sum  Inputs=|+-
  Switch : Switch  Criteria=u2 > Threshold  Threshold=single(pi)  SaturateOnIntegerOverflow=off  InputSameDT=off
  yaw_rate_setpoint : Outport
  wires:
  Bus Element In/1 -> Sum/1
  Bus Element In1/1 -> Sum/2
  Gain/1 -> Saturation/1
  Saturation/1 -> yaw_rate_setpoint/1
  Sum/1 -> Mod/1
  Constant/1 -> Sum1/2, Mod/2
  Mod/1 -> Sum1/1, Switch/3, Switch/2
  Sum1/1 -> Switch/1
  Switch/1 -> Gain/1

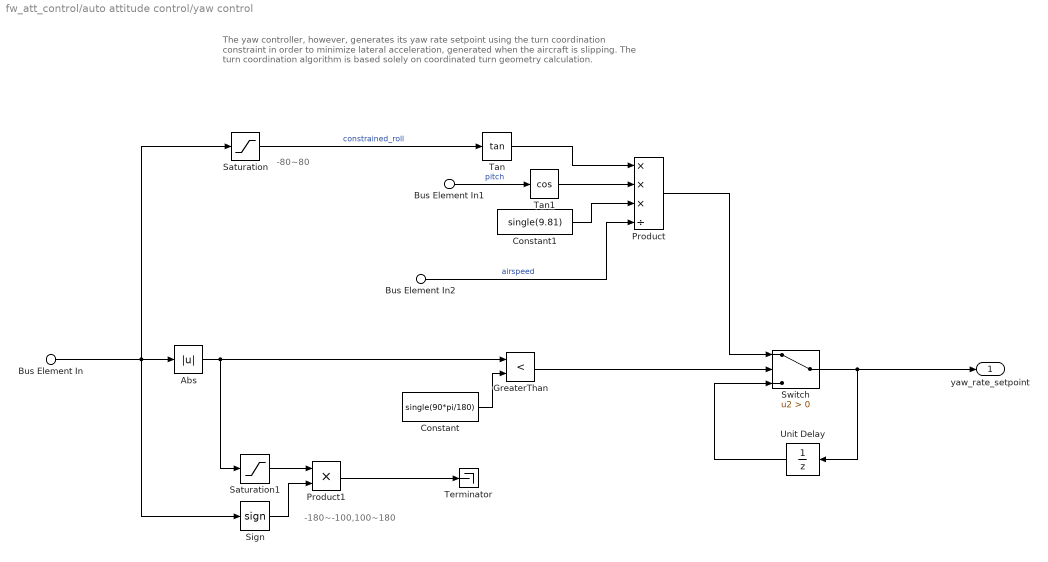
== system fw_att_control/auto attitude control/yaw control ==
  note: The yaw controller, however, generates its yaw rate setpoint using the turn coordination constraint in order to minimize lateral acceleration, generated when the aircraft is slipping. The turn coordination algorithm is based solely on coordinated turn geometry calculation.
  note: -180~-100,100~180
  note: -80~80
  Bus Element In : Inport  PortName=state  Element=roll
  Bus Element In1 : Inport  PortName=state  Element=pitch
  Bus Element In2 : Inport  PortName=state  Element=calibrated_airspeed
  Abs : Abs  SaturateOnIntegerOverflow=off
  Constant : Constant  Value=single(90*pi/180)  OutDataTypeStr=single
  Constant1 : Constant  Value=single(9.81)  OutDataTypeStr=single
  GreaterThan : RelationalOperator  Operator=<  OutDataTypeStr=boolean  RndMeth=Simplest  InputSameDT=off
  Product : Product  Inputs=***/
  Product1 : Product
  Saturation : Saturate  UpperLimit=single(80*pi/180)  LowerLimit=single(-80*pi/180)
  Saturation1 : Saturate  UpperLimit=single(180*pi/180)  LowerLimit=single(100*pi/180)
  Sign : Signum
  Switch : Switch  Criteria=u2 > Threshold  SaturateOnIntegerOverflow=off  InputSameDT=off
  Tan : Trigonometry  Operator=tan
  Tan1 : Trigonometry  Operator=cos
  Terminator : Terminator
  Unit Delay : UnitDelay  SampleTime=-1  HasFrameUpgradeWarning=on
  yaw_rate_setpoint : Outport
  wires:
  Bus Element In/1 -> Sign/1, Saturation/1, Abs/1
  Abs/1 -> Saturation1/1, GreaterThan/1
  Constant/1 -> GreaterThan/2
  Saturation/1 -> Tan/1  "constrained_roll"
  Bus Element In1/1 -> Tan1/1  "pitch"
  Tan/1 -> Product/1
  Tan1/1 -> Product/2
  Constant1/1 -> Product/3
  Bus Element In2/1 -> Product/4  "airspeed"
  Saturation1/1 -> Product1/1
  Sign/1 -> Product1/2
  Product/1 -> Switch/1
  GreaterThan/1 -> Switch/2
  Switch/1 -> yaw_rate_setpoint/1, Unit Delay/1
  Unit Delay/1 -> Switch/3
  Product1/1 -> Terminator/1

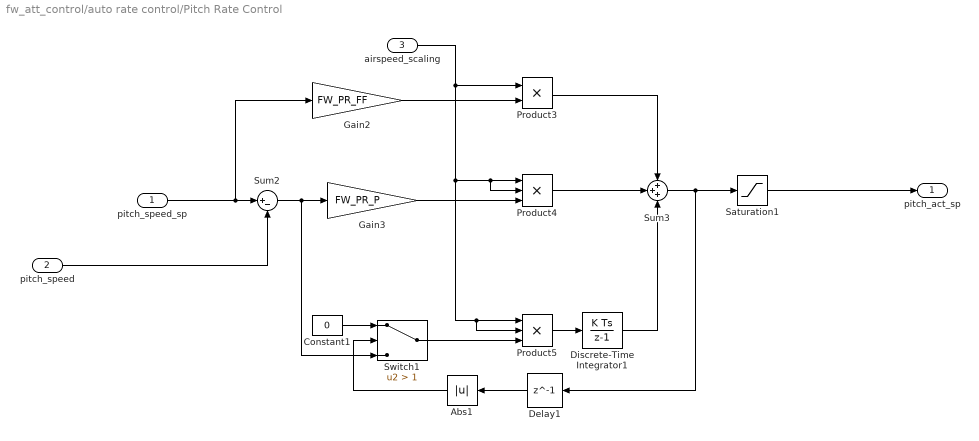
== system fw_att_control/auto rate control/Pitch Rate Control ==
  pitch_speed_sp : Inport
  pitch_speed : Inport  Port=2
  airspeed_scaling : Inport  Port=3
  Abs1 : Abs  SaturateOnIntegerOverflow=off
  Constant1 : Constant  Value=0  OutDataTypeStr=single
  Delay1 : Delay  DelayLength=1
  Discrete-Time Integrator1 : DiscreteIntegrator  gainval=FW_PR_I  SampleTime=-1  LimitOutput=on  UpperSaturationLimit=FW_PR_IMAX  LowerSaturationLimit=-FW_PR_IMAX  ICPrevOutput=DiscIntNeverNeededParam  ICPrevScaledInput=DiscIntNeverNeededParam
  Gain2 : Gain  Gain=FW_PR_FF
  Gain3 : Gain  Gain=FW_PR_P
  Product3 : Product
  Product4 : Product  Inputs=3
  Product5 : Product  Inputs=3
  Saturation1 : Saturate  UpperLimit=1  LowerLimit=-1
  Sum2 : Sum  Inputs=|+-
  Sum3 : Sum  Inputs=3
  Switch1 : Switch  Criteria=u2 > Threshold  Threshold=1  SaturateOnIntegerOverflow=off  InputSameDT=off
  pitch_act_sp : Outport
  wires:
  Delay1/1 -> Abs1/1
  Abs1/1 -> Switch1/2
  Constant1/1 -> Switch1/1
  Product5/1 -> Discrete-Time Integrator1/1
  pitch_speed/1 -> Sum2/2
  Discrete-Time Integrator1/1 -> Sum3/3
  Product3/1 -> Sum3/1
  pitch_speed_sp/1 -> Sum2/1, Gain2/1
  airspeed_scaling/1 -> Product3/1, Product4/1, Product4/2, Product5/2, Product5/1
  Switch1/1 -> Product5/3
  Gain2/1 -> Product3/2
  Sum2/1 -> Gain3/1, Switch1/3
  Gain3/1 -> Product4/3
  Sum3/1 -> Delay1/1, Saturation1/1
  Product4/1 -> Sum3/2
  Saturation1/1 -> pitch_act_sp/1

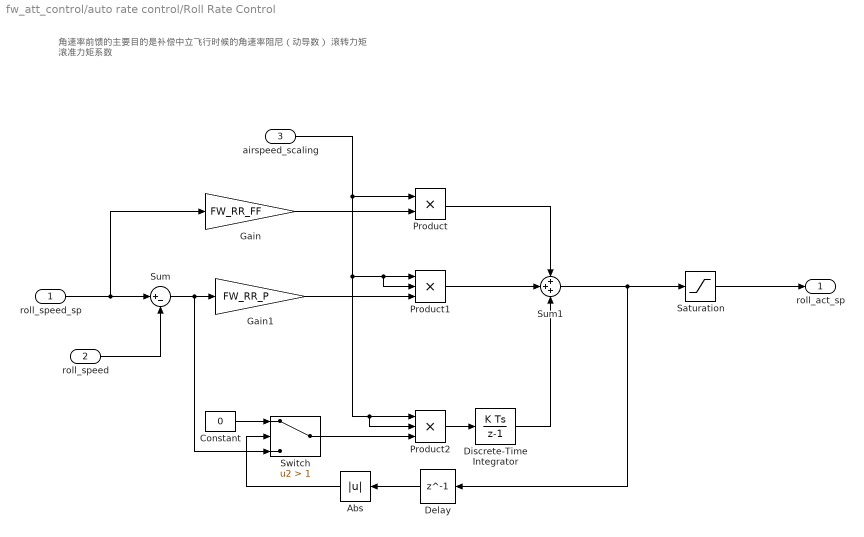
== system fw_att_control/auto rate control/Roll Rate Control ==
  note: 角速率前馈的主要目的是补偿中立飞行时候的角速率阻尼（动导数）
      |
      | 滚转力矩
      | 滚准力矩系数
  roll_speed_sp : Inport
  roll_speed : Inport  Port=2
  airspeed_scaling : Inport  Port=3
  Abs : Abs  SaturateOnIntegerOverflow=off
  Constant : Constant  Value=0  OutDataTypeStr=single
  Delay : Delay  DelayLength=1
  Discrete-Time Integrator : DiscreteIntegrator  gainval=FW_RR_I  SampleTime=-1  LimitOutput=on  UpperSaturationLimit=FW_RR_IMAX  LowerSaturationLimit=-FW_RR_IMAX  ICPrevOutput=DiscIntNeverNeededParam  ICPrevScaledInput=DiscIntNeverNeededParam
  Gain : Gain  Gain=FW_RR_FF
  Gain1 : Gain  Gain=FW_RR_P
  Product : Product
  Product1 : Product  Inputs=3
  Product2 : Product  Inputs=3
  Saturation : Saturate  UpperLimit=1  LowerLimit=-1
  Sum : Sum  Inputs=|+-
  Sum1 : Sum  Inputs=3
  Switch : Switch  Criteria=u2 > Threshold  Threshold=1  SaturateOnIntegerOverflow=off  InputSameDT=off
  roll_act_sp : Outport
  wires:
  Discrete-Time Integrator/1 -> Sum1/3
  Gain/1 -> Product/2
  roll_speed_sp/1 -> Gain/1, Sum/1
  Sum1/1 -> Delay/1, Saturation/1
  Switch/1 -> Product2/3
  Abs/1 -> Switch/2
  Product1/1 -> Sum1/2
  Constant/1 -> Switch/1
  Delay/1 -> Abs/1
  Sum/1 -> Switch/3, Gain1/1
  airspeed_scaling/1 -> Product1/2, Product1/1, Product2/1, Product2/2, Product/1
  Product/1 -> Sum1/1
  Gain1/1 -> Product1/3
  Product2/1 -> Discrete-Time Integrator/1
  roll_speed/1 -> Sum/2
  Saturation/1 -> roll_act_sp/1

== system fw_att_control/auto rate control/Throttle Control ==
  batt_connected : Inport
  batt_scale : Inport  Port=2
  In3 : Inport  Port=3
  Product : Product
  Selector : Selector  InputPortWidth=3  IndexOptions=Index vector (dialog)  Indices=1  OutputSizes=1
  battery scaling : Subsystem
  Out1 : Outport
  wires:
  batt_connected/1 -> battery scaling/1(batt_connected)
  battery scaling/1(battery_scaling) -> Product/1
  Selector/1 -> Product/2
  batt_scale/1 -> battery scaling/2(batt_scale)
  Product/1 -> Out1/1
  In3/1 -> Selector/1

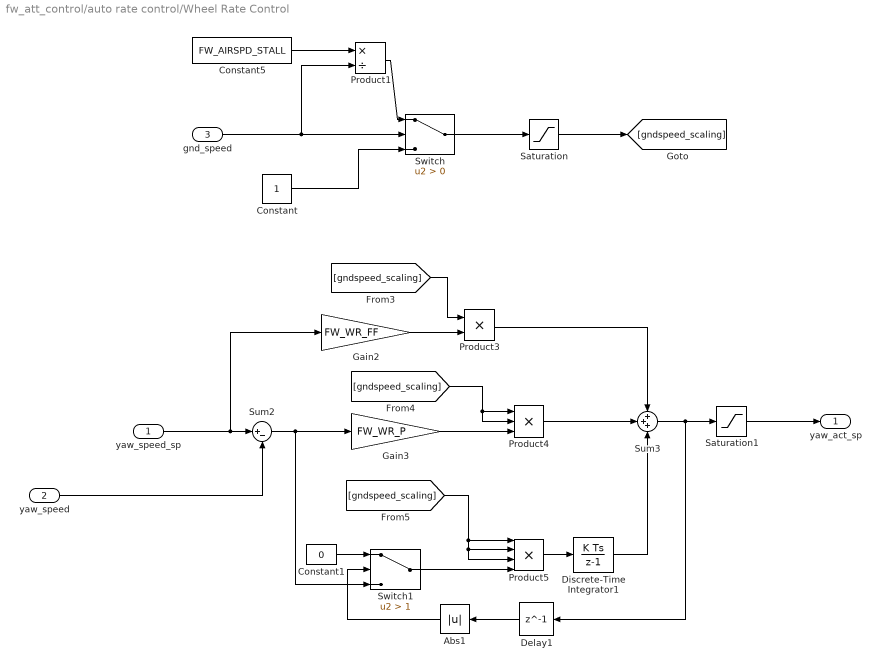
== system fw_att_control/auto rate control/Wheel Rate Control ==
  yaw_speed_sp : Inport
  yaw_speed : Inport  Port=2
  gnd_speed : Inport  Port=3
  Abs1 : Abs  SaturateOnIntegerOverflow=off
  Constant : Constant  OutDataTypeStr=single
  Constant1 : Constant  Value=0  OutDataTypeStr=single
  Constant5 : Constant  Value=FW_AIRSPD_STALL
  Delay1 : Delay  DelayLength=1
  Discrete-Time Integrator1 : DiscreteIntegrator  gainval=FW_WR_I  SampleTime=-1  LimitOutput=on  UpperSaturationLimit=FW_WR_IMAX  LowerSaturationLimit=-FW_WR_IMAX  ICPrevOutput=DiscIntNeverNeededParam  ICPrevScaledInput=DiscIntNeverNeededParam
  Gain2 : Gain  Gain=FW_WR_FF
  Gain3 : Gain  Gain=FW_WR_P
  Product1 : Product  Inputs=*/
  Product3 : Product
  Product4 : Product  Inputs=3
  Product5 : Product  Inputs=4
  Saturation : Saturate  UpperLimit=1  LowerLimit=0
  Saturation1 : Saturate  UpperLimit=1  LowerLimit=-1
  Sum2 : Sum  Inputs=|+-
  Sum3 : Sum  Inputs=3
  Switch : Switch  Criteria=u2 > Threshold  SaturateOnIntegerOverflow=off  InputSameDT=off
  Switch1 : Switch  Criteria=u2 > Threshold  Threshold=1  SaturateOnIntegerOverflow=off  InputSameDT=off
  yaw_act_sp : Outport
  wires:
  Delay1/1 -> Abs1/1
  Abs1/1 -> Switch1/2
  Constant1/1 -> Switch1/1
  Product5/1 -> Discrete-Time Integrator1/1
  yaw_speed/1 -> Sum2/2
  Discrete-Time Integrator1/1 -> Sum3/3
  Product3/1 -> Sum3/1
  [gndspeed_scaling] -> Product4/1, Product4/2
  yaw_speed_sp/1 -> Sum2/1, Gain2/1
  [gndspeed_scaling] -> Product5/2, Product5/3, Product5/1
  Switch1/1 -> Product5/4
  Gain2/1 -> Product3/2
  Saturation1/1 -> yaw_act_sp/1
  Sum2/1 -> Gain3/1, Switch1/3
  [gndspeed_scaling] -> Product3/1
  Gain3/1 -> Product4/3
  Sum3/1 -> Saturation1/1, Delay1/1
  Product4/1 -> Sum3/2
  Saturation/1 -> [gndspeed_scaling]
  Constant5/1 -> Product1/1
  gnd_speed/1 -> Product1/2, Switch/2
  Product1/1 -> Switch/1
  Switch/1 -> Saturation/1
  Constant/1 -> Switch/3

== system fw_att_control/auto rate control/Yaw Rate Control ==
  yaw_speed_sp : Inport
  yaw_speed : Inport  Port=2
  airspeed_scaling : Inport  Port=3
  Abs1 : Abs  SaturateOnIntegerOverflow=off
  Constant1 : Constant  Value=0  OutDataTypeStr=single
  Delay1 : Delay  DelayLength=1
  Discrete-Time Integrator1 : DiscreteIntegrator  gainval=FW_YR_I  SampleTime=-1  LimitOutput=on  UpperSaturationLimit=FW_YR_IMAX  LowerSaturationLimit=-FW_YR_IMAX  ICPrevOutput=DiscIntNeverNeededParam  ICPrevScaledInput=DiscIntNeverNeededParam
  Gain2 : Gain  Gain=FW_YR_FF
  Gain3 : Gain  Gain=FW_YR_P
  Product3 : Product
  Product4 : Product  Inputs=3
  Product5 : Product  Inputs=3
  Saturation1 : Saturate  UpperLimit=1  LowerLimit=-1
  Sum2 : Sum  Inputs=|+-
  Sum3 : Sum  Inputs=3
  Switch1 : Switch  Criteria=u2 > Threshold  Threshold=1  SaturateOnIntegerOverflow=off  InputSameDT=off
  yaw_act_sp : Outport
  wires:
  Product4/1 -> Sum3/2
  Sum3/1 -> Delay1/1, Saturation1/1
  Gain3/1 -> Product4/3
  Sum2/1 -> Switch1/3, Gain3/1
  Gain2/1 -> Product3/2
  Switch1/1 -> Product5/3
  airspeed_scaling/1 -> Product4/2, Product4/1, Product5/1, Product5/2, Product3/1
  yaw_speed_sp/1 -> Gain2/1, Sum2/1
  Product3/1 -> Sum3/1
  Discrete-Time Integrator1/1 -> Sum3/3
  yaw_speed/1 -> Sum2/2
  Product5/1 -> Discrete-Time Integrator1/1
  Constant1/1 -> Switch1/1
  Abs1/1 -> Switch1/2
  Delay1/1 -> Abs1/1
  Saturation1/1 -> yaw_act_sp/1

== system fw_att_control/auto rate control/airspeed scaling ==
  note: /**
      | * Airspeed mode
      | *
      | * For small wings or VTOL without airspeed sensor this parameter can be used to
      | * enable flying without an airspeed reading
      | *
      | * @value 0 Normal (use airspeed if available)
      | * @value 1 Airspeed disabled
      | * @group FW Attitude Control
      | */
  calibrated_airspeed : Inport
  Constant : Constant  Value=FW_ARSP_MODE
  Constant1 : Constant  Value=FW_AIRSPD_TRIM
  Constant2 : Constant  Value=FW_ARSP_SCALE_EN
  Constant3 : Constant  Value=FW_AIRSPD_TRIM
  Constant4 : Constant  OutDataTypeStr=single
  Product : Product  Inputs=*/
  Saturation1 : Saturate  UpperLimit=FW_AIRSPD_MAX  LowerLimit=FW_AIRSPD_STALL
  Saturation3 : Saturate  UpperLimit=1000  LowerLimit=single(0.1)
  Switch : Switch  Criteria=u2 > Threshold  SaturateOnIntegerOverflow=off  InputSameDT=off
  Switch1 : Switch  Criteria=u2 > Threshold  SaturateOnIntegerOverflow=off  InputSameDT=off
  airspeed_scaling : Outport
  wires:
  Switch1/1 -> airspeed_scaling/1
  Switch/1 -> Saturation1/1
  Saturation1/1 -> Saturation3/1
  Constant4/1 -> Switch1/3
  Constant2/1 -> Switch1/2
  Constant/1 -> Switch/2
  Constant1/1 -> Switch/1
  Constant3/1 -> Product/1
  Product/1 -> Switch1/1
  calibrated_airspeed/1 -> Switch/3
  Saturation3/1 -> Product/2  "airspeed_constrained"

== system fw_att_control/auto rate control/Throttle Control/battery scaling ==
  batt_connected : Inport
  batt_scale : Inport  Port=2
  Constant1 : Constant  Value=FW_BAT_SCALE_EN
  Constant2 : Constant  OutDataTypeStr=single
  Constant3 : Constant  OutDataTypeStr=single
  Saturation : Saturate  UpperLimit=inf  LowerLimit=0
  Switch : Switch  Criteria=u2 > Threshold  SaturateOnIntegerOverflow=off  InputSameDT=off
  Switch1 : Switch  Criteria=u2 > Threshold  Threshold=0.5  SaturateOnIntegerOverflow=off  InputSameDT=off
  battery_scaling : Outport
  wires:
  Constant2/1 -> Switch/3
  Switch/1 -> battery_scaling/1
  batt_scale/1 -> Saturation/1
  Saturation/1 -> Switch1/1
  batt_connected/1 -> Switch1/2
  Switch1/1 -> Switch/1
  Constant1/1 -> Switch/2
  Constant3/1 -> Switch1/3

== stateflow chart fw_att_control/Subsystem/Chart ==
  (default) -> (junction 2) : {
      | manual_attitude_control=0;
      | manual_rate_control =0;
      | manual_actuator_control=0;
      | }
  (junction 2) -> (junction 13) [order 2]
  (junction 2) -> (junction 4) [order 1] : [manual_enabled]
  (junction 13) -> (junction 15)
  (junction 4) -> (junction 7) [order 2]
  (junction 4) -> (junction 1) [order 1] : [~climb_rate_enabled]
  (junction 7) -> (junction 24)
  (junction 1) -> (junction 55) [order 1] : [attitude_enabled]
  (junction 1) -> (junction 11) [order 2] : [rates_enabled]
  (junction 55) -> (junction 57) : {manual_attitude_control=1;}
  (junction 1) -> (junction 20) [order 3] : {manual_actuator_control=0;}
  (junction 11) -> (junction 17) : {manual_rate_control=1;}
  (junction 57) -> (junction 20)
  (junction 17) -> (junction 20)
  (junction 20) -> (junction 27)
  (junction 24) -> (junction 27)
  (junction 27) -> (junction 61)
  (junction 15) -> (junction 61)
  (junction 61) -> (junction 64)
  data: manual_attitude_control output; manual_rate_control output; manual_enabled input; climb_rate_enabled input; attitude_enabled input; rates_enabled input; manual_actuator_control output
